simulink model "car"  (R2018a)
settings: Solver=ode5  StartTime=0.0  StopTime=450  FixedStep=0.3  RelTol=1e-3
undefined symbols (not defined in the file): sigbuilder_block
libraries: fuzblock x1
settings Model: Creator=doanduy  LastModifiedBy=DELL
settings DataIOCC: ReturnWorkspaceOutputs=on
settings SFSimCC: SimUseLocalCustomCode=on
settings RTWCC: RTWUseLocalCustomCode=on

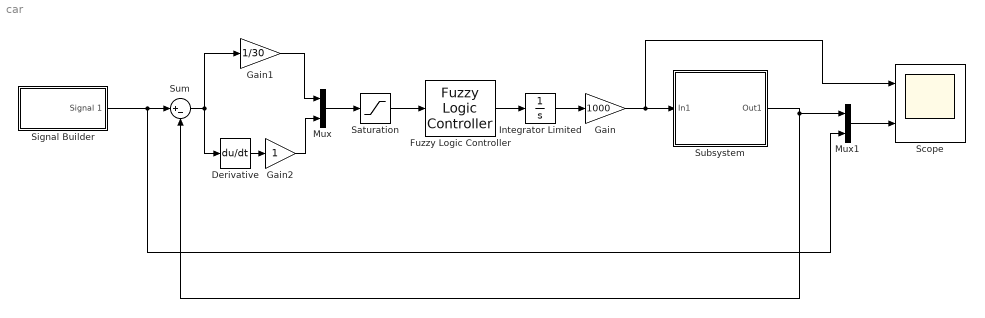
== system car ==
  Derivative : Derivative
  Fuzzy Logic Controller : fuzblock/Fuzzy Logic  Controller  FIS='fuzzy1.fis'  OutputSampleNumber=101  DataType=double  FuzzifiedInputs=off  RuleFiringStrengths=off  RuleOutputs=off  AggregatedOutputs=off  SimulateUsing=Interpreted execution  OutOfRangeInputValueMessage=warning  NoRuleFiredMessage=warning  EmptyOutputFuzzySetMessage=warning
  Gain : Gain  Gain=1000
  Gain1 : Gain  Gain=1/30
  Gain2 : Gain
  Integrator Limited : Integrator  LimitOutput=on  UpperSaturationLimit=1  LowerSaturationLimit=-1
  Mux : Mux  Inputs=2
  Mux1 : Mux  Inputs=2
  Saturation : Saturate  UpperLimit=1  LowerLimit=-1
  Scope : Scope  NumInputPorts=2
  Signal Builder : Subsystem  Tag=STV Subsys  LoadFcn=sigbuilder_block('load');  StartFcn=sigbuilder_block('start');  StopFcn=sigbuilder_block('stop');  ClipboardFcn=sigbuilder_block('clipboard');  mask(Sigbuilder block){tuvar=[0:10]}
      mask help: Simulink:masks:SigbuilderBlock_MD
      mask init:
      | if ~strcmp(get_param(bdroot(gcbh),'SimulationStatus'),'stopped') tuvar = sigbuilder_block('maskInit'); end
      settings: CopyFcn=sigbuilder_block('copy');  DeleteFcn=sigbuilder_block('delete');  ModelCloseFcn=sigbuilder_block('modelClose');  PreSaveFcn=sigbuilder_block('preSave');  PauseFcn=sigbuilder_block('pause');  ContinueFcn=sigbuilder_block('continue');  NameChangeFcn=sigbuilder_block('namechange');  OpenFcn=sigbuilder_block('open',[5.4 5.4 1141.2 580.8 ]);  CloseFcn=sigbuilder_block('close');
      mask Display: plot(0, 0, 100, 100,[2, 2, 32, 32, 2], [68, 8, 8, 68, 68],[32, 2], [38, 38], [32, 19, 2],[53, 60, 44], [32, 17, 17, 2],[16, 16, 31, 31]);txt = getActiveGroup(gcbh);text(2, 100, txt,'verticalAlignment', 'top');
  Subsystem : Subsystem
  Sum : Sum  Inputs=|+-
  wires:
  Gain/1 -> Scope/1, Subsystem/1(In1)
  Integrator Limited/1 -> Gain/1
  Signal Builder/1(Signal 1) -> Mux1/2, Sum/1
  Sum/1 -> Gain1/1, Derivative/1
  Derivative/1 -> Gain2/1
  Fuzzy Logic Controller/1 -> Integrator Limited/1
  Gain2/1 -> Mux/2
  Gain1/1 -> Mux/1
  Mux/1 -> Saturation/1
  Saturation/1 -> Fuzzy Logic Controller/1
  Subsystem/1(Out1) -> Mux1/1, Sum/2
  Mux1/1 -> Scope/2

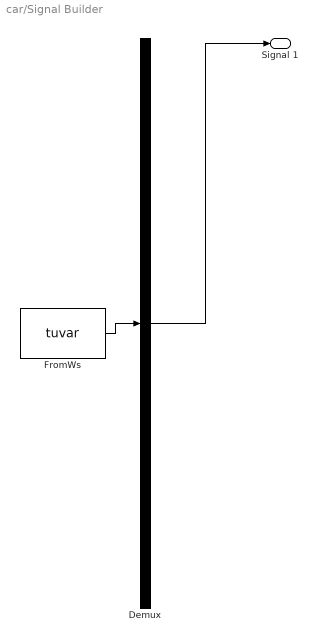
== system car/Signal Builder ==
  Demux : Demux  Tag=STV Demux  Outputs=1
  FromWs : FromWorkspace  Tag=STV FromWs  VariableName=tuvar  SampleTime=0
      SigBuilderData=|
      | common.afterFinalStr = 'Extrapolate'
      | common.sampleTime = 0
      | dataSet.timeRange = [0 450]
      | dataSet.name = 'Group 1'
      | sbobj.Groups.Name = 'Group 1'
      | sbobj.Groups.Signals.Name = 'Signal 1'
      | sbobj.Groups.Signals.XData = [0 103 103 164.5 164.5 233.5 233.5 305.5 305.5 379 379 450]
      | sbobj.Groups.Signals.YData = [30 30 20 20 10 10 25 25 15 15 30 30]
      | sbobj.Groups.TimeRange = [0 450]
  Signal 1 : Outport  Tag=STV Outport  VectorParamsAs1DForOutWhenUnconnected=on
  wires:
  Demux/1 -> Signal 1/1
  FromWs/1 -> Demux/1

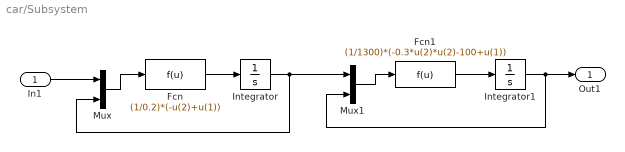
== system car/Subsystem ==
  In1 : Inport
  Fcn : Fcn  Expr=(1/0.2)*(-u(2)+u(1))
  Fcn1 : Fcn  Expr=(1/1300)*(-0.3*u(2)*u(2)-100+u(1))
  Integrator : Integrator  LimitOutput=on  UpperSaturationLimit=1000  LowerSaturationLimit=-1000
  Integrator1 : Integrator  InitialCondition=15  LimitOutput=on  UpperSaturationLimit=30  LowerSaturationLimit=0
  Mux : Mux  Inputs=2
  Mux1 : Mux  Inputs=2
  Out1 : Outport  VectorParamsAs1DForOutWhenUnconnected=on
  wires:
  In1/1 -> Mux/1
  Mux/1 -> Fcn/1
  Fcn/1 -> Integrator/1
  Integrator/1 -> Mux1/1, Mux/2
  Fcn1/1 -> Integrator1/1
  Integrator1/1 -> Mux1/2, Out1/1
  Mux1/1 -> Fcn1/1
